simulink model "SAR_logic"  (R2018b)
settings: Solver=VariableStepAuto  StartTime=0.0  StopTime=39  RelTol=1e-3
libraries: simulink_extras x36
settings Model: Creator=iamcy  LastModifiedBy=iamcy

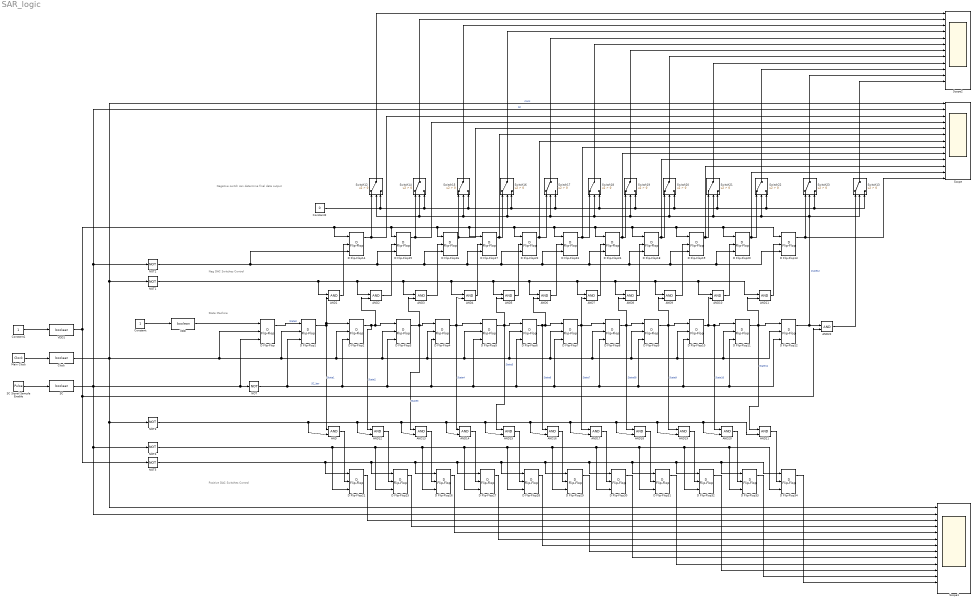
== system SAR_logic ==
  note: Negative switch can determine final data output
  note: Neg DAC Switches Control
  note: State Machine
  note: Positive DAC Switches Control
  AND{,1..22} (23 alike) : Logic  IconShape=distinctive  AllPortsSameDT=off  OutDataTypeStr=boolean
  Clock : DataTypeConversion  OutDataTypeStr=boolean
  Constant : Constant
  Constant1 : Constant
  Constant2 : Constant  Value=0
  D Flip-Flop{,1..34} (35 alike) : simulink_extras/Flip Flops/D Flip-Flop
      settings: SourceProductName=Simulink
  Main Clock : simulink_extras/Flip Flops/Clock  period=1
  NOT{,1..5} (6 alike) : Logic  Operator=NOT  IconShape=distinctive  AllPortsSameDT=off  OutDataTypeStr=boolean
  SC : DataTypeConversion  OutDataTypeStr=boolean
  SC Signal Sample Enable : DiscretePulseGenerator  PulseType=Time based  Period=13  PulseWidth=100/13
  Scope : Scope  NumInputPorts=13
  Scope1 : Scope  NumInputPorts=14
  Scope2 : Scope  NumInputPorts=13
  Switch{12..23} (12 alike) : Switch  Criteria=u2 > Threshold
  VDD : DataTypeConversion  OutDataTypeStr=boolean
  VDD1 : DataTypeConversion  OutDataTypeStr=boolean
  wires:
  D Flip-Flop/1 -> D Flip-Flop1/1  "State0"
  D Flip-Flop2/1 -> AND12/1, AND2/2, D Flip-Flop3/1  "State2"
  D Flip-Flop1/1 -> AND/1, AND1/2, D Flip-Flop2/1  "State1"
  Constant/1 -> VDD/1
  Main Clock/1 -> Clock/1
  SC Signal Sample Enable/1 -> SC/1
  SC/1 -> Scope/2, NOT2/1, D Flip-Flop/3, NOT/1, Scope1/2, NOT4/1  "SC"
  VDD/1 -> D Flip-Flop/1
  D Flip-Flop4/1 -> AND14/1, AND4/2, D Flip-Flop5/1  "State4"
  D Flip-Flop5/1 -> AND15/1, AND5/2, D Flip-Flop6/1  "State5"
  D Flip-Flop6/1 -> AND6/2, D Flip-Flop7/1, AND16/1  "State6"
  NOT/1 -> D Flip-Flop4/3, D Flip-Flop6/3, D Flip-Flop8/3, D Flip-Flop11/3, D Flip-Flop12/3, D Flip-Flop10/3, D Flip-Flop9/3, D Flip-Flop7/3, D Flip-Flop5/3, D Flip-Flop3/3, D Flip-Flop2/3, D Flip-Flop1/3  "SC_bar"
  Clock/1 -> D Flip-Flop/2, D Flip-Flop1/2, D Flip-Flop3/2, D Flip-Flop4/2, D Flip-Flop5/2, D Flip-Flop6/2, D Flip-Flop7/2, D Flip-Flop8/2, D Flip-Flop11/2, D Flip-Flop12/2, D Flip-Flop10/2, D Flip-Flop9/2, D Flip-Flop2/2, NOT3/1, Scope1/1, Scope/1, NOT1/1  "clock"
  D Flip-Flop3/1 -> AND13/1, D Flip-Flop4/1, AND3/2  "State3"
  D Flip-Flop7/1 -> AND17/1, D Flip-Flop8/1, AND7/2  "State7"
  D Flip-Flop8/1 -> AND8/2, AND18/1, D Flip-Flop9/1  "State08"
  D Flip-Flop9/1 -> AND19/1, AND9/2, D Flip-Flop10/1  "State9"
  D Flip-Flop10/1 -> AND10/2, AND20/1, D Flip-Flop11/1  "State10"
  D Flip-Flop11/1 -> AND21/1, D Flip-Flop12/1, AND11/2  "State11"
  Constant1/1 -> VDD1/1
  VDD1/1 -> D Flip-Flop14/1, D Flip-Flop13/1, D Flip-Flop20/1, D Flip-Flop19/1, D Flip-Flop18/1, D Flip-Flop24/1, D Flip-Flop23/1, D Flip-Flop22/1, D Flip-Flop17/1, D Flip-Flop16/1, D Flip-Flop15/1, NOT5/1, AND22/2
  NOT1/1 -> AND11/1, AND10/1, AND9/1, AND8/1, AND7/1, AND6/1, AND5/1, AND4/1, AND3/1, AND2/1, AND1/1
  AND1/1 -> D Flip-Flop14/2
  AND2/1 -> D Flip-Flop15/2
  AND3/1 -> D Flip-Flop16/2
  AND4/1 -> D Flip-Flop17/2
  AND5/1 -> D Flip-Flop22/2
  AND6/1 -> D Flip-Flop23/2
  AND7/1 -> D Flip-Flop24/2
  AND8/1 -> D Flip-Flop18/2
  AND9/1 -> D Flip-Flop19/2
  AND10/1 -> D Flip-Flop20/2
  AND11/1 -> D Flip-Flop13/2
  NOT2/1 -> D Flip-Flop13/3, D Flip-Flop20/3, D Flip-Flop19/3, D Flip-Flop18/3, D Flip-Flop24/3, D Flip-Flop23/3, D Flip-Flop22/3, D Flip-Flop17/3, D Flip-Flop16/3, D Flip-Flop15/3, D Flip-Flop14/3
  NOT4/1 -> D Flip-Flop21/3, D Flip-Flop25/3, D Flip-Flop26/3, D Flip-Flop27/3, D Flip-Flop28/3, D Flip-Flop29/3, D Flip-Flop30/3, D Flip-Flop31/3, D Flip-Flop32/3, D Flip-Flop33/3, D Flip-Flop34/3
  AND/1 -> D Flip-Flop21/2
  NOT3/1 -> AND/2, AND12/2, AND13/2, AND14/2, AND15/2, AND16/2, AND17/2, AND18/2, AND19/2, AND21/2, AND20/2
  AND12/1 -> D Flip-Flop25/2
  AND13/1 -> D Flip-Flop26/2
  AND14/1 -> D Flip-Flop27/2
  AND15/1 -> D Flip-Flop28/2
  AND16/1 -> D Flip-Flop29/2
  AND17/1 -> D Flip-Flop30/2
  AND18/1 -> D Flip-Flop31/2
  AND19/1 -> D Flip-Flop32/2
  AND20/1 -> D Flip-Flop33/2
  AND21/1 -> D Flip-Flop34/2
  NOT5/1 -> D Flip-Flop34/1, D Flip-Flop33/1, D Flip-Flop32/1, D Flip-Flop31/1, D Flip-Flop30/1, D Flip-Flop29/1, D Flip-Flop28/1, D Flip-Flop27/1, D Flip-Flop26/1, D Flip-Flop25/1, D Flip-Flop21/1
  D Flip-Flop12/1 -> Switch12/2, Switch14/2, Switch15/2, Switch16/2, Switch17/2, Switch18/2, Switch19/2, Switch20/2, Switch21/2, Switch22/2, Switch13/2, Switch23/2, AND22/1  "state12"
  AND22/1 -> Switch13/1
  D Flip-Flop13/1 -> Scope/13, Switch23/1
  D Flip-Flop14/1 -> Scope/3, Switch12/1
  D Flip-Flop15/1 -> Scope/4, Switch14/1
  D Flip-Flop16/1 -> Scope/5, Switch15/1
  D Flip-Flop17/1 -> Switch16/1, Scope/6
  D Flip-Flop22/1 -> Switch17/1, Scope/7
  D Flip-Flop23/1 -> Scope/8, Switch18/1
  D Flip-Flop24/1 -> Scope/9, Switch19/1
  D Flip-Flop18/1 -> Scope/10, Switch20/1
  D Flip-Flop19/1 -> Scope/11, Switch21/1
  D Flip-Flop20/1 -> Scope/12, Switch22/1
  Constant2/1 -> Switch13/3, Switch23/3, Switch22/3, Switch21/3, Switch20/3, Switch19/3, Switch18/3, Switch17/3, Switch16/3, Switch15/3, Switch14/3, Switch12/3
  Switch12/1 -> Scope2/1
  Switch14/1 -> Scope2/2
  Switch15/1 -> Scope2/3
  Switch16/1 -> Scope2/4
  Switch17/1 -> Scope2/5
  Switch18/1 -> Scope2/6
  Switch19/1 -> Scope2/7
  Switch20/1 -> Scope2/8
  Switch21/1 -> Scope2/9
  Switch22/1 -> Scope2/10
  Switch23/1 -> Scope2/11
  Switch13/1 -> Scope2/12
  D Flip-Flop21/1 -> Scope1/3
  D Flip-Flop25/1 -> Scope1/4
  D Flip-Flop26/1 -> Scope1/5
  D Flip-Flop27/1 -> Scope1/6
  D Flip-Flop28/1 -> Scope1/7
  D Flip-Flop29/1 -> Scope1/8
  D Flip-Flop30/1 -> Scope1/9
  D Flip-Flop31/1 -> Scope1/10
  D Flip-Flop32/1 -> Scope1/11
  D Flip-Flop33/1 -> Scope1/12
  D Flip-Flop34/1 -> Scope1/13
